simulink model "WuerfelPIModel_SIM"  (R2017b)
settings: Solver=FixedStepAuto  StartTime=0.0  StopTime=31.5  FixedStep=0.001  RelTol=1e-3
values from neighbouring files (symbols this model uses):
  K1 = (g * mK*l_AC+mR*l_AB)/IK    (= 57.1105052634)    [ParameterInit.m]    (also in WuerfelParameter.mat = 26.5237013135; WuerfelParameterIdentification.m = K(1))
  K2 = Cphi/IK    (= 1.80492803577)    [ParameterInit.m]    (also in WuerfelParameter.mat = 0.524765473269; WuerfelParameterIdentification.m = K(2))
  phi_0 = phi(1)    [ParameterInit.m]
  uK_0 = uk(1)    [ParameterInit.m]
undefined symbols (not defined in the file or in its folder): magnitude
settings Model: Creator=michael  LastModifiedBy=michael

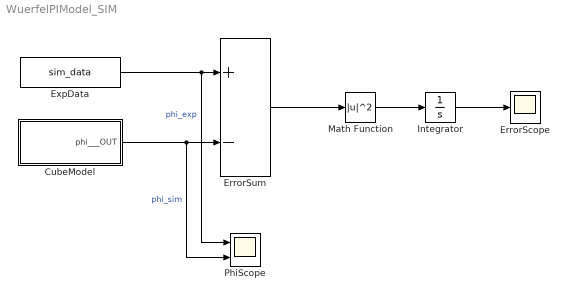
== system WuerfelPIModel_SIM ==
  CubeModel : Subsystem
  ErrorScope : Scope
  ErrorSum : Sum  Inputs=+-
  ExpData : FromWorkspace  VariableName=sim_data  SampleTime=0
  Integrator : Integrator
  Math Function : Math  Operator=magnitude^2  SaturateOnIntegerOverflow=on
  PhiScope : Scope  NumInputPorts=2
  wires:
  CubeModel/1(phi___OUT) -> PhiScope/2, ErrorSum/2  "phi_sim"
  ExpData/1 -> PhiScope/1, ErrorSum/1  "phi_exp"
  ErrorSum/1 -> Math Function/1
  Math Function/1 -> Integrator/1
  Integrator/1 -> ErrorScope/1

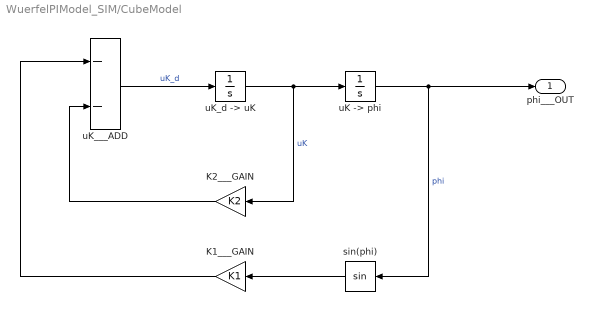
== system WuerfelPIModel_SIM/CubeModel ==
  K1___GAIN : Gain  Gain=K1
  K2___GAIN : Gain  Gain=K2
  sin(phi) : Trigonometry
  "uK -> phi" : Integrator  InitialCondition=phi_0
  uK___ADD : Sum  Inputs=--
  "uK_d -> uK" : Integrator  InitialCondition=uK_0
  phi___OUT : Outport
  wires:
  uK___ADD/1 -> "uK_d -> uK"/1  "uK_d"
  "uK_d -> uK"/1 -> K2___GAIN/1, "uK -> phi"/1  "uK"
  "uK -> phi"/1 -> sin(phi)/1, phi___OUT/1  "phi"
  sin(phi)/1 -> K1___GAIN/1
  K1___GAIN/1 -> uK___ADD/1
  K2___GAIN/1 -> uK___ADD/2
